simulink model "mainmodel"  (R2020a)
settings: Solver=VariableStepAuto  StartTime=0.0  StopTime=10.0  RelTol=1e-3
settings Model: Creator=Bhanu  LastModifiedBy=Bhanu

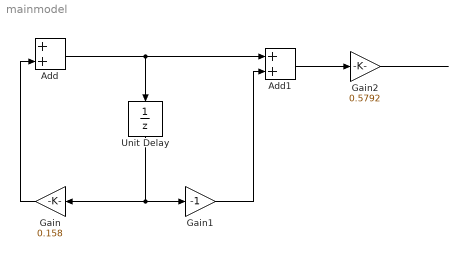
== system mainmodel ==
  Add : Sum
  Add1 : Sum
  Gain : Gain  Gain=0.158
  Gain1 : Gain  Gain=-1
  Gain2 : Gain  Gain=0.5792
  Unit Delay : UnitDelay  SampleTime=-1  HasFrameUpgradeWarning=on
  wires:
  Add/1 -> Add1/1, Unit Delay/1
  Unit Delay/1 -> Gain1/1, Gain/1
  Gain/1 -> Add/2
  Gain1/1 -> Add1/2
  Add1/1 -> Gain2/1
  Gain2/1 -> ?
  ? -> Add/1
